simulink model "RNN_Node"  (R2020b)
settings: Solver=VariableStepAuto  StartTime=0.0  StopTime=10.0  RelTol=1e-3
settings Model: Creator=chank  LastModifiedBy=chank

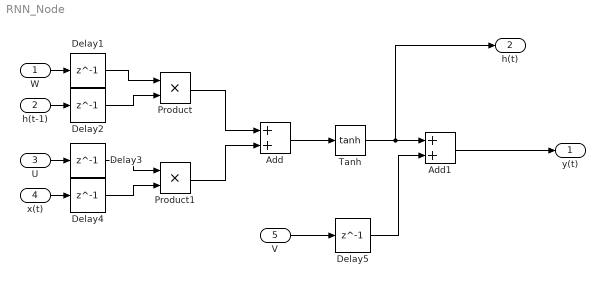
== system RNN_Node ==
  W : Inport  OutDataTypeStr=single
  h(t-1) : Inport  Port=2  OutDataTypeStr=single
  U : Inport  Port=3  OutDataTypeStr=single
  x(t) : Inport  Port=4  OutDataTypeStr=single
  V : Inport  Port=5  OutDataTypeStr=single
  Add : Sum
  Add1 : Sum
  Delay{1..5} (5 alike) : Delay  DelayLength=1
  Product : Product
  Product1 : Product
  Tanh : Trigonometry  Operator=tanh
  y(t) : Outport
  h(t) : Outport  Port=2
  wires:
  Add/1 -> Tanh/1
  Product/1 -> Add/1
  Product1/1 -> Add/2
  Tanh/1 -> h(t)/1, Add1/1
  W/1 -> Delay1/1
  h(t-1)/1 -> Delay2/1
  U/1 -> Delay3/1
  x(t)/1 -> Delay4/1
  Delay1/1 -> Product/1
  Delay2/1 -> Product/2
  Delay3/1 -> Product1/1
  Delay4/1 -> Product1/2
  V/1 -> Delay5/1
  Delay5/1 -> Add1/2
  Add1/1 -> y(t)/1
